simulink model "RM3"  (R2014b)
settings: Solver=ode4  StartTime=0  StopTime=400  FixedStep=0.001  RelTol=1e-3
undefined symbols (not defined in the file or in its folder): body, constraint, pto
libraries: PTOSim_Lib x6, WECSim_Lib x5
settings Model: SimulationMode=rapid-accelerator  Creator=mlawson  LastModifiedBy=sor
settings SolverCC: AlgebraicLoopSolver=LineSearch
settings DataIOCC: LimitDataPoints=off  SaveOutput=off  SaveTime=off
settings DebuggingCC: UnderspecifiedInitializationDetection=Classic  MergeDetectMultiDrivingBlocksExec=none  StateNameClashWarn=warning
settings ExplorerConfigSet: InternalSimMechanicsExplorerSettings="<ExplorerConfiguration><canonicalview>default</canonicalview><TilePanel><TileInfo><Tiles Columns=\"1\" Count=\"1\" Rows=\"1\"><Column Left=\"2\" Weight=\"1\"/><Column Left=\"1335\"/><Row Top=\"2\" Weight=\"1\"/><Row Top=\"911\"/><Tile Height=\"1\" Width=\"1\" X=\"0\" Y=\"0\"/></Tiles></TileInfo><SceneInfo><SceneViewer><BGColor><R>0.60000002384185791</R><G>0.60000002384185791</G><B>0.60000002384185791</B></BGColor><Camera><Position><X>365.37645888990272</X><Y>-369.82486814446582</Y><Z>359.64809521743916</Z></Position><Center><X>-6.7351450971904585</X><Y>2.2867358426280204</Y><Z>-12.463508769654169</Z></Center><Up><X>-0.40824829046386307</X><Y>0.40824829046386307</Y><Z>0.81649658092772615</Z></Up><Left>-57.820127362122818</Left><Right>57.820127362122818</Right><Bottom>-38.308817187253304</Bottom><Top>38.308817187253304</Top></Camera></SceneViewer></SceneInfo></TilePanel></ExplorerConfiguration>"

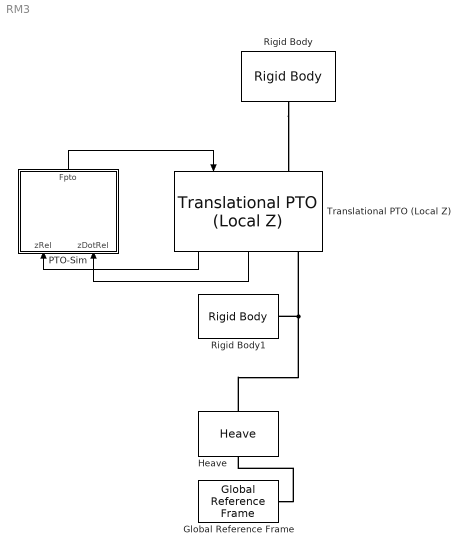
== system RM3 ==
  Global Reference Frame : WECSim_Lib/Frames/Global Reference Frame  waves=waves  simu=simu
  Heave : WECSim_Lib/Constraints/Heave  constraint=constraint(1)
      settings: AttributesFormatString=%<constraint>
  PTO-Sim : Subsystem  mask{Parameter1=0}
      mask prompts: Parameter1 "pto"
  Rigid Body : WECSim_Lib/Body Elements/Rigid Body  body=body(1)
      settings: AttributesFormatString=%<body>
  Rigid Body1 : WECSim_Lib/Body Elements/Rigid Body  body=body(2)
      settings: AttributesFormatString=%<body>
  Translational PTO (Local Z) : WECSim_Lib/PTOs/Translational PTO  (Local Z)  pto=pto(1)
      settings: AttributesFormatString=%<pto>
  wires:
  PTO-Sim/1(Fpto) -> Translational PTO (Local Z)/1
  Translational PTO (Local Z)/2 -> PTO-Sim/2(zDotRel)
  Translational PTO (Local Z)/1 -> PTO-Sim/1(zRel)
  connections:
  Global Reference Frame/RConn1 -- Heave/LConn1
  Heave/RConn1 -- Rigid Body1/RConn1 -- Translational PTO (Local Z)/RConn1
  Rigid Body/RConn1 -- Translational PTO (Local Z)/LConn1

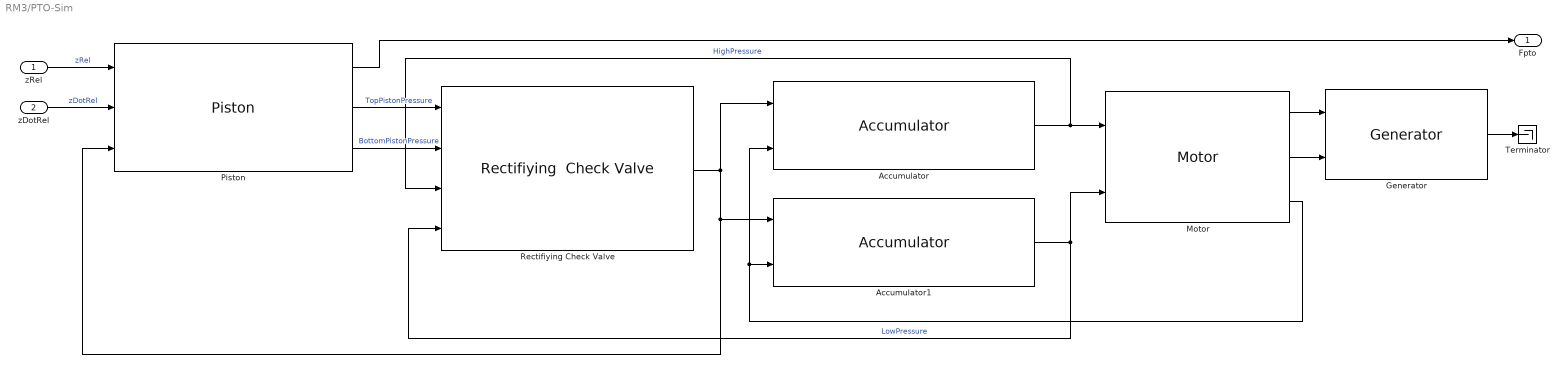
== system RM3/PTO-Sim ==
  zRel : Inport
  zDotRel : Inport  Port=2
  Accumulator : PTOSim_Lib/Hydraulic_PTO/Accumulator  OverrideUsingVariant=Variant  pto=0
  Accumulator1 : PTOSim_Lib/Hydraulic_PTO/Accumulator  OverrideUsingVariant=Variant1  pto=0
  Generator : PTOSim_Lib/Hydraulic_PTO/Generator  pto=0
  "Motor " : PTOSim_Lib/Hydraulic_PTO/Motor   pto=0
  "Piston " : PTOSim_Lib/Hydraulic_PTO/Piston    pto=0
  Rectifiying Check Valve : PTOSim_Lib/Hydraulic_PTO/Rectifiying  Check Valve  pto=0
  Terminator : Terminator
  Fpto : Outport
  wires:
  zRel/1 -> "Piston "/1  "zRel"
  zDotRel/1 -> "Piston "/2  "zDotRel"
  "Piston "/2 -> Rectifiying Check Valve/1  "TopPistonPressure"
  "Piston "/3 -> Rectifiying Check Valve/2  "BottomPistonPressure"
  "Motor "/1 -> Generator/1
  "Motor "/2 -> Generator/2
  "Motor "/3 -> Accumulator/2, Accumulator1/2
  Accumulator/1 -> Rectifiying Check Valve/3, "Motor "/1  "HighPressure"
  Accumulator1/1 -> "Motor "/2, Rectifiying Check Valve/4  "LowPressure"
  Rectifiying Check Valve/1 -> "Piston "/3, Accumulator1/1, Accumulator/1
  Generator/1 -> Terminator/1
  "Piston "/1 -> Fpto/1
